simulink model "filter_1_10"  (Simulink 7.8)
settings: Solver=ode23  StartTime=0.0  StopTime=10.0  RelTol=10e-3
libraries: dsparch4 x5, dspsigops x3
settings Model: Creator=svenhoffmann  LastModifiedBy=josef  ExtModeAutoUpdateStatusClock=off
settings SolverCC: ConsecutiveZCsStepRelTol=auto
settings DataIOCC: SignalLoggingName=sigsOut
settings OptimizationCC: InitFltsAndDblsToZero=on
settings DebuggingCC: SaveWithParameterizedLinksMsg=none  SignalResolutionControl=TryResolveAllWithWarning  SolverPrmCheckMsg=none  MultiTaskDSMMsg=warning  MultiTaskCondExecSysMsg=none  FcnCallInpInsideContextMsg=Use local settings  StrictBusMsg=None
settings HardwareCC: TargetUnknown=on
settings RTWCC: IncludeERTFirstTime=on
settings GRTTargetCC: TargetFcnLib=ansi_tfl_tmw.mat

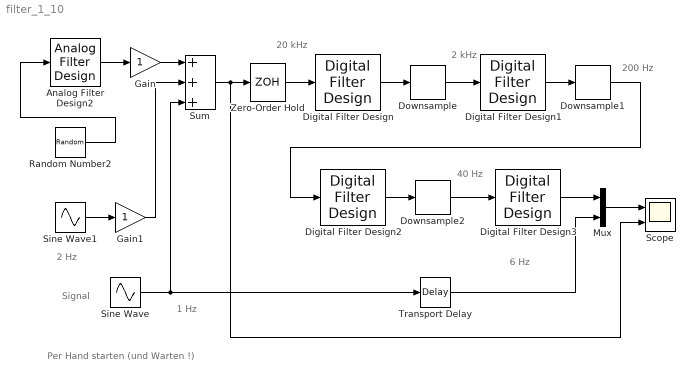
== system filter_1_10 ==
  note: 20 kHz
  note: 2 kHz
  note: 200 Hz
  note: 40 Hz
  note: 6 Hz
  note: 1 Hz
  note: Signal
  note: 2 Hz
  note: Per Hand starten (und Warten !)
  Analog Filter Design2 : dsparch4/Analog Filter Design  method=Chebyshev I  filttype=Bandpass  N=8  Wlo=2*pi*100  Whi=2*pi*5000  Rp=2  Rs=40
  Digital Filter Design{,1..3} (4 alike) : dsparch4/Digital Filter Design  mwdsp_browser_bugfix_var=off
  Downsample : dspsigops/Downsample  N=10  phase=0  InputProcessing=Inherited (this choice will be removed - see release notes)  RateOptions=Enforce single-rate processing  smode=Allow multirate  fmode=Maintain input frame size  ic=0
  Downsample1 : dspsigops/Downsample  N=10  phase=0  InputProcessing=Inherited (this choice will be removed - see release notes)  RateOptions=Enforce single-rate processing  smode=Allow multirate  fmode=Maintain input frame size  ic=0
  Downsample2 : dspsigops/Downsample  N=5  phase=0  InputProcessing=Inherited (this choice will be removed - see release notes)  RateOptions=Enforce single-rate processing  smode=Allow multirate  fmode=Maintain input frame size  ic=0
  Gain : Gain  SaturateOnIntegerOverflow=on  OutDataTypeStr=Inherit: Same as input  ParamDataTypeStr=Inherit: Same as input
  Gain1 : Gain  SaturateOnIntegerOverflow=on  OutDataTypeStr=Inherit: Same as input  ParamDataTypeStr=Inherit: Same as input
  Mux : Mux  Inputs=2
  Random Number2 : RandomNumber  SampleTime=0
  Scope : Scope  NumInputPorts=2
      settings: TimeRange=5  YMin=-1~-2  YMax=1~2  MaxDataPoints=100000
  Sine Wave : Sin  Frequency=2*pi*1  SampleTime=0
  Sine Wave1 : Sin  Frequency=2*pi*2  SampleTime=0
  Sum : Sum  Inputs=+++  SaturateOnIntegerOverflow=on
  Transport Delay : TransportDelay  DelayTime=0.51
  Zero-Order Hold : ZeroOrderHold  SampleTime=1/20000
  wires:
  Sine Wave/1 -> Sum/3, Transport Delay/1
  Random Number2/1 -> Analog Filter Design2/1
  Analog Filter Design2/1 -> Gain/1
  Gain/1 -> Sum/1
  Sum/1 -> Zero-Order Hold/1, Scope/2
  Digital Filter Design/1 -> Downsample/1
  Downsample/1 -> Digital Filter Design1/1
  Digital Filter Design1/1 -> Downsample1/1
  Digital Filter Design2/1 -> Downsample2/1
  Downsample1/1 -> Digital Filter Design2/1
  Zero-Order Hold/1 -> Digital Filter Design/1
  Downsample2/1 -> Digital Filter Design3/1
  Digital Filter Design3/1 -> Mux/1
  Mux/1 -> Scope/1
  Transport Delay/1 -> Mux/2
  Gain1/1 -> Sum/2
  Sine Wave1/1 -> Gain1/1
